simulink model "com_serie_speed"  (R2017a)
settings: Solver=VariableStepAuto  StartTime=0.0  StopTime=1  RelTol=1e-3
undefined symbols (not defined in the file): serial
libraries: instrumentlib x2
settings Model: Creator=Martin  LastModifiedBy=Martin

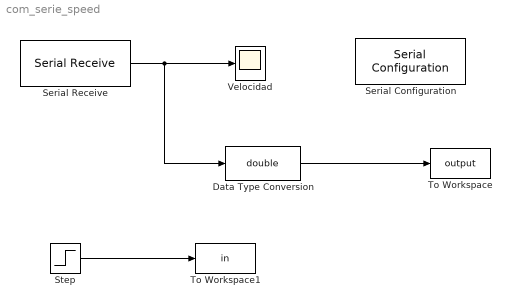
== system com_serie_speed ==
  Data Type Conversion : DataTypeConversion  OutDataTypeStr=double
  Serial Configuration : instrumentlib/Serial Configuration  Priority=-200000  ComPortMenu=<Please select a port...>  ComPort=COM4  ObjConstructor=serial('COM4');  BaudRate=9600  DataBits=8  Parity=none  StopBits=1  FlowControl=none  Timeout=10  ByteOrder=LittleEndian
  Serial Receive : instrumentlib/Serial Receive  ComPortMenu=<Please select a port...>  ComPort=COM4  ObjConstructor=serial('COM4');  Terminator=<none>  DataSize="[1  1]"  DataType=single  EnableBlockingMode=on  ActionDataUnavailable=Output last received value  CustomValue=0  SampleTime=0.01
  Step : Step  Time=0  After=4875  SampleTime=0.01
  To Workspace : ToWorkspace  VariableName=output  SaveFormat=Structure With Time  SampleTime=0.01
      settings: Save2DSignal=2-D array (concatenate along first dimension)
  To Workspace1 : ToWorkspace  VariableName=in  SaveFormat=Structure With Time  SampleTime=0.01
      settings: Save2DSignal=2-D array (concatenate along first dimension)
  Velocidad : Scope
  wires:
  Serial Receive/1 -> Data Type Conversion/1, Velocidad/1
  Data Type Conversion/1 -> To Workspace/1
  Step/1 -> To Workspace1/1
